simulink model "PRO_TestHarness"  (Simulink 8.6)
settings: Solver=ode45  StartTime=0.0  StopTime=10.0  RelTol=1e-3
PreLoadFcn:
  | addpath('./Workspace/')
  | load('./Workspace/EnvVar.mat')
  | if exist('tl_preloadfcn','file'), tl_preloadfcn(gcs,402); end
PostLoadFcn:
  | if exist('tl_postloadfcn','file'), tl_postloadfcn(gcs,402); end
InitFcn:
  | if exist('tlds_init','file'), tlds_init(gcs); end
StartFcn:
  | if exist('tlds_start','file'), tlds_start(gcs); end
StopFcn:
  | if exist('tlds_stop','file'), tlds_stop(gcs); end
undefined symbols (not defined in the file or in its folder): ddv, sigbuilder_block, Ts
libraries: tllib x19, simulink x2
(part 5 of 5)

== system PRO_TestHarness/PRO_AC_ProductionCycles/Subsystem/PRO_AC_ProductionCycles/PRO_AC_ProductionCycles/PRO_runProductionCycles/PRO enabled/FctTrigAbortCycle_AllPRO/For Iterator Subsystem/Algo PRO/FctTrigg_PRO ==
  bPreConditionsCommonFlag : Inport
  bPreActivation_PRO_in : Inport  Port=2
  Function : tllib/Function  data={'stepfunctionname','TriggerPRO','stepfunctionclass','STATIC_FCN_ASR4','codecomment',['This function is in charge of' char(10) 'providing the following outputs:' char(10) '' char(10) '- Trigger flag for PRO1 cycle' char(10) '- Pre Activation flag for PRO1 cycle' char(10) '- Pre Conditions flag for PRO1 cycle' char(10) '- Triggering Source for PRO1 cycle' char(10) '' char(10) 'according to the inputs:' char(10) '' char(10) '- executed cycle number' char(10) '- consistent cycle requested by diagnostic' char(10) '- common PRO preconditions flag'],'module','PRO_AC_ProductionCycles','date',736463.55395115737}  displayString=FUNCTION
  ToFormatFlag_PreActivationFlag : Subsystem
  ToFormatFlag_PreConditionsFlag : Subsystem
  ToFormatFlag_TriggeringOrder : Subsystem
  ToFormat_TriggeringSource : Subsystem
  bTriggeringOrder_Tester_PRO : Logic  AllPortsSameDT=off  OutDataTypeStr=boolean  mask(TL_LogicalOperator){data={'output',{'name','$B'},'date',735626.4046887384}}
      settings: DeleteFcn=if exist('delete_tlblock','file')==2,delete_tlblock(gcbh);end  NameChangeFcn=if exist('rename_tlblock','file')==2,rename_tlblock(gcbh);end  OpenFcn=if exist('tl_open_blockdlg','file')==2,tl_open_blockdlg(gcbh);else,open_system(gcbh,'parameter');end
      mask Help: eval(['if exist(''tl_online_help'',''file'') == 2, tl_online_help(''Topic'',''TL_LogicalOperator''),else, web([''jar:file:///'',matlabroot,''/help/toolbox/simulink/help.jar!/slref/' lower(get_param(gcbh,'Blocktype')) '.html''], ''-helpbrowser''),end'])
      mask Display: plot([-0.05, 1.05, NaN, -0.05, 1.05],[.01, .01, NaN, .99, .99])
  b8TriggeringOrder : Outport  PortDimensions=1
  b8PreActivationFlag : Outport  Port=2  PortDimensions=1
  b8PreConditionsFlag : Outport  Port=3  PortDimensions=1
  u8TriggeringSource_output : Outport  Port=4  PortDimensions=1
  wires:
  ToFormatFlag_TriggeringOrder/1(Out1) -> b8TriggeringOrder/1
  [bPreConditionsCommonFlag] -> ToFormatFlag_PreConditionsFlag/1(In1), bTriggeringOrder_Tester_PRO/1
  ToFormatFlag_PreConditionsFlag/1(Out1) -> b8PreConditionsFlag/1
  bTriggeringOrder_Tester_PRO/1 -> ToFormat_TriggeringSource/1(In1), ToFormatFlag_TriggeringOrder/1(In1)
  bPreConditionsCommonFlag/1 -> [bPreConditionsCommonFlag]
  ToFormatFlag_PreActivationFlag/1(Out2) -> b8PreActivationFlag/1
  ToFormat_TriggeringSource/1(Out1) -> u8TriggeringSource_output/1
  [bPreActivation_PRO] -> bTriggeringOrder_Tester_PRO/2
  [bPreActivation_PRO] -> ToFormatFlag_PreActivationFlag/1(In1)
  bPreActivation_PRO_in/1 -> [bPreActivation_PRO]

== system PRO_TestHarness/PRO_AC_ProductionCycles/Subsystem/PRO_AC_ProductionCycles/PRO_AC_ProductionCycles/PRO_runProductionCycles/PRO enabled/FctCommonPROManageInputs/FctCommonEvaluatePreActivationFlags/For Iterator Subsystem/FctEvaluatePreActivationFlags_PRO/Acquite Diag Request From DIA ==
  Action Port : ActionPort  ActionType=then
  ClearDiagRequestCycle : Subsystem  RequirementInfo={} %GIDa_6c044e8f_69a0_4de9_90b7_cd2120bfe9b6  TreatAsAtomicUnit=on

== system PRO_TestHarness/PRO_AC_ProductionCycles/Subsystem/PRO_AC_ProductionCycles/PRO_AC_ProductionCycles/PRO_runProductionCycles/PRO enabled/FctCommonPROManageInputs/FctCommonEvaluatePreActivationFlags/For Iterator Subsystem/FctEvaluatePreActivationFlags_PRO/Clear activation ==
  In1 : Inport
  Action Port : ActionPort  ActionType=elseif
  Out1 : Outport
  wires:
  In1/1 -> Out1/1

== system PRO_TestHarness/PRO_AC_ProductionCycles/Subsystem/PRO_AC_ProductionCycles/PRO_AC_ProductionCycles/PRO_runProductionCycles/PRO enabled/FctCommonPROManageInputs/FctCommonEvaluatePreActivationFlags/For Iterator Subsystem/FctEvaluatePreActivationFlags_PRO/Keep activation ==
  In1 : Inport
  Action Port : ActionPort  ActionType=else
  Out1 : Outport
  wires:
  In1/1 -> Out1/1

== system PRO_TestHarness/PRO_AC_ProductionCycles/Subsystem/PRO_AC_ProductionCycles/PRO_AC_ProductionCycles/PRO_runProductionCycles/PRO enabled/FctCommonPROManageInputs/FctCommonEvaluatePreActivationFlags/For Iterator Subsystem/FctEvaluatePreActivationFlags_PRO/Set activation ==
  In1 : Inport
  Action Port : ActionPort  ActionType=then
  Out1 : Outport
  wires:
  In1/1 -> Out1/1

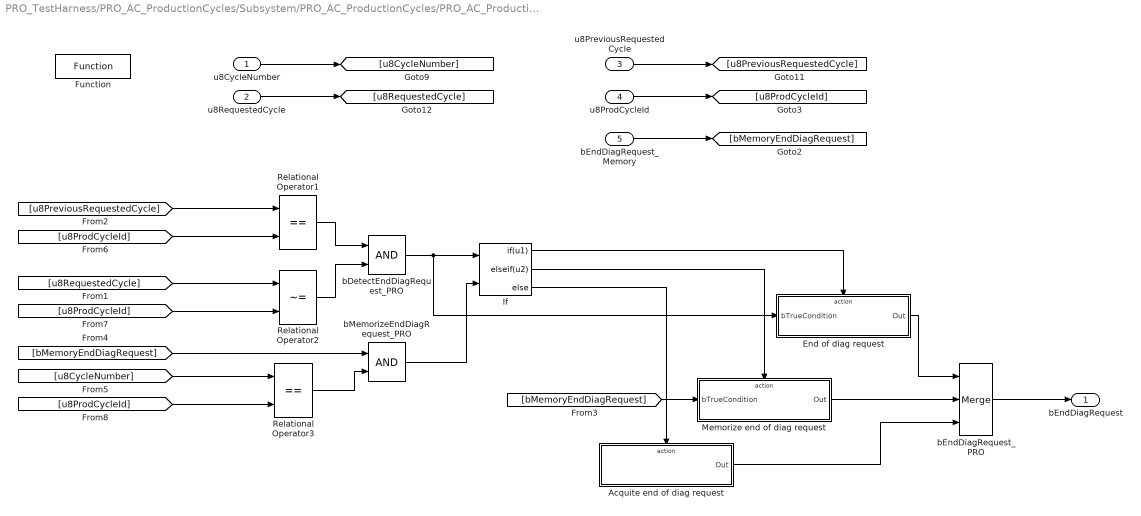
== system PRO_TestHarness/PRO_AC_ProductionCycles/Subsystem/PRO_AC_ProductionCycles/PRO_AC_ProductionCycles/PRO_runProductionCycles/PRO enabled/FctTrigAbortCycle_AllPRO/For Iterator Subsystem/Algo PRO/FctAbort_PRO/Check end diag request for PRO ==
  u8CycleNumber : Inport  PortDimensions=1
  u8RequestedCycle : Inport  Port=2  OutDataTypeStr=uint8  PortDimensions=1
  u8PreviousRequestedCycle : Inport  Port=3  OutDataTypeStr=uint8  PortDimensions=1
  u8ProdCycleId : Inport  Port=4  PortDimensions=1
  bEndDiagRequest_Memory : Inport  Port=5  PortDimensions=1
  Acquite end of diag request : Subsystem  TreatAsAtomicUnit=on
  End of diag request : Subsystem  TreatAsAtomicUnit=on
  Function : tllib/Function  data={'stepfunctionname','DetectEndOfDiagRequestPRO','stepfunctionclass','STATIC_FCN_ASR4','codecomment',['This function is in charge of' char(10) 'providing the following outputs:' char(10) '' char(10) '- End flag in case of PRO1 diagnostic request' char(10) '' char(10) 'according to the inputs:' char(10) '' char(10) '- executed cycle number' char(10) '- consistent cycle requested by diagnostic' char(10) '- previous (10 ms before) consistent cycle requested by diagnostic'],'module','PRO_AC_ProductionCycles','date',736463.55394269677}  displayString=FUNCTION
  If : If  NumInputs=2  IfExpression=u1  ElseIfExpressions=u2
  Memorize end of diag request : Subsystem  TreatAsAtomicUnit=on
  Relational Operator1 : RelationalOperator  Operator===  OutDataTypeStr=boolean  mask(TL_RelationalOperator){data={'date',735679.60375327547}}
      settings: DeleteFcn=if exist('delete_tlblock','file')==2,delete_tlblock(gcbh);end  NameChangeFcn=if exist('rename_tlblock','file')==2,rename_tlblock(gcbh);end  OpenFcn=if exist('tl_open_blockdlg','file')==2,tl_open_blockdlg(gcbh);else,open_system(gcbh,'parameter');end
      mask Help: eval(['if exist(''tl_online_help'',''file'') == 2, tl_online_help(''Topic'',''TL_RelationalOperator''),else, web([''jar:file:///'',matlabroot,''/help/toolbox/simulink/help.jar!/slref/' lower(get_param(gcbh,'Blocktype')) '.html''], ''-helpbrowser''),end'])
      mask Display: plot([-0.05, 1.05, NaN, -0.05, 1.05],[.01, .01, NaN, .99, .99])
  Relational Operator2 : RelationalOperator  Operator=~=  OutDataTypeStr=boolean  mask(TL_RelationalOperator){data={'date',735679.60375291668}}
      settings: DeleteFcn=if exist('delete_tlblock','file')==2,delete_tlblock(gcbh);end  NameChangeFcn=if exist('rename_tlblock','file')==2,rename_tlblock(gcbh);end  OpenFcn=if exist('tl_open_blockdlg','file')==2,tl_open_blockdlg(gcbh);else,open_system(gcbh,'parameter');end
      mask Help: eval(['if exist(''tl_online_help'',''file'') == 2, tl_online_help(''Topic'',''TL_RelationalOperator''),else, web([''jar:file:///'',matlabroot,''/help/toolbox/simulink/help.jar!/slref/' lower(get_param(gcbh,'Blocktype')) '.html''], ''-helpbrowser''),end'])
      mask Display: plot([-0.05, 1.05, NaN, -0.05, 1.05],[.01, .01, NaN, .99, .99])
  Relational Operator3 : RelationalOperator  Operator===  OutDataTypeStr=boolean  mask(TL_RelationalOperator){data={'date',735679.60375273146}}
      settings: DeleteFcn=if exist('delete_tlblock','file')==2,delete_tlblock(gcbh);end  NameChangeFcn=if exist('rename_tlblock','file')==2,rename_tlblock(gcbh);end  OpenFcn=if exist('tl_open_blockdlg','file')==2,tl_open_blockdlg(gcbh);else,open_system(gcbh,'parameter');end
      mask Help: eval(['if exist(''tl_online_help'',''file'') == 2, tl_online_help(''Topic'',''TL_RelationalOperator''),else, web([''jar:file:///'',matlabroot,''/help/toolbox/simulink/help.jar!/slref/' lower(get_param(gcbh,'Blocktype')) '.html''], ''-helpbrowser''),end'])
      mask Display: plot([-0.05, 1.05, NaN, -0.05, 1.05],[.01, .01, NaN, .99, .99])
  bDetectEndDiagRequest_PRO : Logic  AllPortsSameDT=off  OutDataTypeStr=boolean  mask(TL_LogicalOperator){data={'output',{'name','$B'},'date',735679.60375237267}}
      settings: DeleteFcn=if exist('delete_tlblock','file')==2,delete_tlblock(gcbh);end  NameChangeFcn=if exist('rename_tlblock','file')==2,rename_tlblock(gcbh);end  OpenFcn=if exist('tl_open_blockdlg','file')==2,tl_open_blockdlg(gcbh);else,open_system(gcbh,'parameter');end
      mask Help: eval(['if exist(''tl_online_help'',''file'') == 2, tl_online_help(''Topic'',''TL_LogicalOperator''),else, web([''jar:file:///'',matlabroot,''/help/toolbox/simulink/help.jar!/slref/' lower(get_param(gcbh,'Blocktype')) '.html''], ''-helpbrowser''),end'])
      mask Display: plot([-0.05, 1.05, NaN, -0.05, 1.05],[.01, .01, NaN, .99, .99])
  bEndDiagRequest_PRO : Merge  Inputs=3  InitialOutput=0  mask(TL_Merge){data={'output',{'name','$B','type','Bool','inheritscaling',0},'date',735679.60375219909}}
      settings: CopyFcn=if exist('tl_reset_reviewflag','file')==2,tl_reset_reviewflag(gcbh);end  DeleteFcn=if exist('delete_tlblock','file')==2,delete_tlblock(gcbh);end  NameChangeFcn=if exist('rename_tlblock','file')==2,rename_tlblock(gcbh);end  OpenFcn=if exist('tl_open_blockdlg','file')==2,tl_open_blockdlg(gcbh);else,open_system(gcbh,'parameter');end
      mask Help: eval(['if exist(''tl_online_help'',''file'') == 2, tl_online_help(''Topic'',''TL_Merge''),else, web([''jar:file:///'',matlabroot,''/help/toolbox/simulink/help.jar!/slref/' lower(get_param(gcbh,'Blocktype')) '.html''], ''-helpbrowser''),end'])
      mask Display: plot([-0.05, 1.05, NaN, -0.05, 1.05],[.01, .01, NaN, .99, .99])
  bMemorizeEndDiagRequest_PRO : Logic  AllPortsSameDT=off  OutDataTypeStr=boolean  mask(TL_LogicalOperator){data={'output',{'name','$B'},'date',735679.60375165509}}
      settings: DeleteFcn=if exist('delete_tlblock','file')==2,delete_tlblock(gcbh);end  NameChangeFcn=if exist('rename_tlblock','file')==2,rename_tlblock(gcbh);end  OpenFcn=if exist('tl_open_blockdlg','file')==2,tl_open_blockdlg(gcbh);else,open_system(gcbh,'parameter');end
      mask Help: eval(['if exist(''tl_online_help'',''file'') == 2, tl_online_help(''Topic'',''TL_LogicalOperator''),else, web([''jar:file:///'',matlabroot,''/help/toolbox/simulink/help.jar!/slref/' lower(get_param(gcbh,'Blocktype')) '.html''], ''-helpbrowser''),end'])
      mask Display: plot([-0.05, 1.05, NaN, -0.05, 1.05],[.01, .01, NaN, .99, .99])
  bEndDiagRequest : Outport  PortDimensions=1
  wires:
  [u8ProdCycleId] -> Relational Operator1/2
  [u8PreviousRequestedCycle] -> Relational Operator1/1
  Relational Operator1/1 -> bDetectEndDiagRequest_PRO/1
  [u8RequestedCycle] -> Relational Operator2/1
  [u8ProdCycleId] -> Relational Operator2/2
  Relational Operator2/1 -> bDetectEndDiagRequest_PRO/2
  bDetectEndDiagRequest_PRO/1 -> If/1, End of diag request/1(bTrueCondition)
  If/1 -> End of diag request/Action
  End of diag request/1(Out) -> bEndDiagRequest_PRO/1
  Memorize end of diag request/1(Out) -> bEndDiagRequest_PRO/2
  Acquite end of diag request/1(Out) -> bEndDiagRequest_PRO/3
  If/2 -> Memorize end of diag request/Action
  If/3 -> Acquite end of diag request/Action
  [bMemoryEndDiagRequest] -> Memorize end of diag request/1(bTrueCondition)
  [u8CycleNumber] -> Relational Operator3/1
  [u8ProdCycleId] -> Relational Operator3/2
  [bMemoryEndDiagRequest] -> bMemorizeEndDiagRequest_PRO/1
  bMemorizeEndDiagRequest_PRO/1 -> If/2
  Relational Operator3/1 -> bMemorizeEndDiagRequest_PRO/2
  bEndDiagRequest_PRO/1 -> bEndDiagRequest/1
  u8CycleNumber/1 -> [u8CycleNumber]
  u8RequestedCycle/1 -> [u8RequestedCycle]
  u8PreviousRequestedCycle/1 -> [u8PreviousRequestedCycle]
  u8ProdCycleId/1 -> [u8ProdCycleId]
  bEndDiagRequest_Memory/1 -> [bMemoryEndDiagRequest]

== system PRO_TestHarness/PRO_AC_ProductionCycles/Subsystem/PRO_AC_ProductionCycles/PRO_AC_ProductionCycles/PRO_runProductionCycles/PRO enabled/FctTrigAbortCycle_AllPRO/For Iterator Subsystem/Algo PRO/FctAbort_PRO/ToFormatFlag_bInterruptFlag ==
  In1 : Inport
  If Action Subsystem4 : Subsystem  TreatAsAtomicUnit=on
  If Action Subsystem5 : Subsystem  TreatAsAtomicUnit=on
  If2 : If  IfExpression=u1
  b8ComputedInterruptFlag : Merge  InitialOutput=[ddv('RTE_DEFINES/KB8_ALGO_FLAG_OFF')]  mask(TL_Merge){data={'output',{'type','UInt8','inheritscaling',0},'date',736811.34356223384}}
      settings: CopyFcn=if exist('tl_reset_reviewflag') == 2, tl_reset_reviewflag(gcbh); end  DeleteFcn=if exist('delete_tlblock','file')==2,delete_tlblock(gcbh);end  NameChangeFcn=if exist('rename_tlblock','file')==2,rename_tlblock(gcbh);end  OpenFcn=if exist('tl_open_blockdlg','file')==2,tl_open_blockdlg(gcbh);else,open_system(gcbh,'parameter');end
      mask Help: eval(['if exist(''tl_online_help'',''file'') == 2, tl_online_help(''Topic'',''TL_Merge''),else, web([''jar:file:///'',matlabroot,''/help/toolbox/simulink/help.jar!/slref/' lower(get_param(gcbh,'Blocktype')) '.html''], ''-helpbrowser''),end'])
      mask Display: plot([-0.05, 1.05, NaN, -0.05, 1.05],[.01, .01, NaN, .99, .99])
  b8NewInterruptFlag_PRO : Gain  OutDataTypeStr=uint8  mask(TL_Gain){data={'output',{'name','$B','type','UInt8'},'date',735664.46096548613}}
      settings: CopyFcn=if exist('tl_reset_reviewflag') == 2, tl_reset_reviewflag(gcbh); end  DeleteFcn=if exist('delete_tlblock','file')==2,delete_tlblock(gcbh);end  NameChangeFcn=if exist('rename_tlblock','file')==2,rename_tlblock(gcbh);end  OpenFcn=if exist('tl_open_blockdlg','file')==2,tl_open_blockdlg(gcbh);else,open_system(gcbh,'parameter');end
      mask Help: eval(['if exist(''tl_online_help'',''file'') == 2, tl_online_help(''Topic'',''TL_Gain''),else, web([''jar:file:///'',matlabroot,''/help/toolbox/simulink/help.jar!/slref/' lower(get_param(gcbh,'Blocktype')) '.html''], ''-helpbrowser''),end'])
      mask Display: plot([0, .9, 0],[.05, .5, .95])
  Out1 : Outport
  wires:
  If2/1 -> If Action Subsystem4/Action
  b8ComputedInterruptFlag/1 -> b8NewInterruptFlag_PRO/1
  If Action Subsystem4/1(Out) -> b8ComputedInterruptFlag/1
  If Action Subsystem5/1(Out) -> b8ComputedInterruptFlag/2
  If2/2 -> If Action Subsystem5/Action
  In1/1 -> If2/1
  b8NewInterruptFlag_PRO/1 -> Out1/1

== system PRO_TestHarness/PRO_AC_ProductionCycles/Subsystem/PRO_AC_ProductionCycles/PRO_AC_ProductionCycles/PRO_runProductionCycles/PRO enabled/FctTrigAbortCycle_AllPRO/For Iterator Subsystem/Algo PRO/FctTrigg_PRO/ToFormatFlag_PreActivationFlag ==
  In1 : Inport
  If : If  IfExpression=u1
  If Action Subsystem : Subsystem  TreatAsAtomicUnit=on
  If Action Subsystem1 : Subsystem  TreatAsAtomicUnit=on
  b8NewPreActivationFlag_PRO : Gain  OutDataTypeStr=uint8  mask(TL_Gain){data={'output',{'name','$B','type','UInt8'},'date',735661.6408991667}}
      settings: CopyFcn=if exist('tl_reset_reviewflag') == 2, tl_reset_reviewflag(gcbh); end  DeleteFcn=if exist('delete_tlblock','file')==2,delete_tlblock(gcbh);end  NameChangeFcn=if exist('rename_tlblock','file')==2,rename_tlblock(gcbh);end  OpenFcn=if exist('tl_open_blockdlg','file')==2,tl_open_blockdlg(gcbh);else,open_system(gcbh,'parameter');end
      mask Help: eval(['if exist(''tl_online_help'',''file'') == 2, tl_online_help(''Topic'',''TL_Gain''),else, web([''jar:file:///'',matlabroot,''/help/toolbox/simulink/help.jar!/slref/' lower(get_param(gcbh,'Blocktype')) '.html''], ''-helpbrowser''),end'])
      mask Display: plot([0, .9, 0],[.05, .5, .95])
  b8PreActivationFlag_PRO : Merge  InitialOutput=[ddv('RTE_DEFINES/KB8_ALGO_FLAG_OFF')]  mask(TL_Merge){data={'output',{'type','UInt8','inheritscaling',0},'date',736811.34117243055}}
      settings: CopyFcn=if exist('tl_reset_reviewflag') == 2, tl_reset_reviewflag(gcbh); end  DeleteFcn=if exist('delete_tlblock','file')==2,delete_tlblock(gcbh);end  NameChangeFcn=if exist('rename_tlblock','file')==2,rename_tlblock(gcbh);end  OpenFcn=if exist('tl_open_blockdlg','file')==2,tl_open_blockdlg(gcbh);else,open_system(gcbh,'parameter');end
      mask Help: eval(['if exist(''tl_online_help'',''file'') == 2, tl_online_help(''Topic'',''TL_Merge''),else, web([''jar:file:///'',matlabroot,''/help/toolbox/simulink/help.jar!/slref/' lower(get_param(gcbh,'Blocktype')) '.html''], ''-helpbrowser''),end'])
      mask Display: plot([-0.05, 1.05, NaN, -0.05, 1.05],[.01, .01, NaN, .99, .99])
  Out2 : Outport
  wires:
  If/1 -> If Action Subsystem/Action
  b8PreActivationFlag_PRO/1 -> b8NewPreActivationFlag_PRO/1
  If Action Subsystem/1(Out) -> b8PreActivationFlag_PRO/1
  If Action Subsystem1/1(Out) -> b8PreActivationFlag_PRO/2
  If/2 -> If Action Subsystem1/Action
  In1/1 -> If/1
  b8NewPreActivationFlag_PRO/1 -> Out2/1

== system PRO_TestHarness/PRO_AC_ProductionCycles/Subsystem/PRO_AC_ProductionCycles/PRO_AC_ProductionCycles/PRO_runProductionCycles/PRO enabled/FctTrigAbortCycle_AllPRO/For Iterator Subsystem/Algo PRO/FctTrigg_PRO/ToFormatFlag_PreConditionsFlag ==
  In1 : Inport
  If Action Subsystem4 : Subsystem  TreatAsAtomicUnit=on
  If Action Subsystem5 : Subsystem  TreatAsAtomicUnit=on
  If2 : If  IfExpression=u1
  b8ComputedPreConditionsFlag : Merge  InitialOutput=[ddv('RTE_DEFINES/KB8_ALGO_FLAG_OFF')]  mask(TL_Merge){data={'output',{'type','UInt8','inheritscaling',0},'date',736811.341286632}}
      settings: CopyFcn=if exist('tl_reset_reviewflag') == 2, tl_reset_reviewflag(gcbh); end  DeleteFcn=if exist('delete_tlblock','file')==2,delete_tlblock(gcbh);end  NameChangeFcn=if exist('rename_tlblock','file')==2,rename_tlblock(gcbh);end  OpenFcn=if exist('tl_open_blockdlg','file')==2,tl_open_blockdlg(gcbh);else,open_system(gcbh,'parameter');end
      mask Help: eval(['if exist(''tl_online_help'',''file'') == 2, tl_online_help(''Topic'',''TL_Merge''),else, web([''jar:file:///'',matlabroot,''/help/toolbox/simulink/help.jar!/slref/' lower(get_param(gcbh,'Blocktype')) '.html''], ''-helpbrowser''),end'])
      mask Display: plot([-0.05, 1.05, NaN, -0.05, 1.05],[.01, .01, NaN, .99, .99])
  b8NewPreConditionsFlag_PRO : Gain  OutDataTypeStr=uint8  mask(TL_Gain){data={'output',{'name','$B','type','UInt8'},'date',735661.64106355328}}
      settings: CopyFcn=if exist('tl_reset_reviewflag') == 2, tl_reset_reviewflag(gcbh); end  DeleteFcn=if exist('delete_tlblock','file')==2,delete_tlblock(gcbh);end  NameChangeFcn=if exist('rename_tlblock','file')==2,rename_tlblock(gcbh);end  OpenFcn=if exist('tl_open_blockdlg','file')==2,tl_open_blockdlg(gcbh);else,open_system(gcbh,'parameter');end
      mask Help: eval(['if exist(''tl_online_help'',''file'') == 2, tl_online_help(''Topic'',''TL_Gain''),else, web([''jar:file:///'',matlabroot,''/help/toolbox/simulink/help.jar!/slref/' lower(get_param(gcbh,'Blocktype')) '.html''], ''-helpbrowser''),end'])
      mask Display: plot([0, .9, 0],[.05, .5, .95])
  Out1 : Outport
  wires:
  If2/1 -> If Action Subsystem4/Action
  b8ComputedPreConditionsFlag/1 -> b8NewPreConditionsFlag_PRO/1
  If Action Subsystem4/1(Out) -> b8ComputedPreConditionsFlag/1
  If Action Subsystem5/1(Out) -> b8ComputedPreConditionsFlag/2
  If2/2 -> If Action Subsystem5/Action
  In1/1 -> If2/1
  b8NewPreConditionsFlag_PRO/1 -> Out1/1

== system PRO_TestHarness/PRO_AC_ProductionCycles/Subsystem/PRO_AC_ProductionCycles/PRO_AC_ProductionCycles/PRO_runProductionCycles/PRO enabled/FctTrigAbortCycle_AllPRO/For Iterator Subsystem/Algo PRO/FctTrigg_PRO/ToFormatFlag_TriggeringOrder ==
  In1 : Inport
  If : If  IfExpression=u1
  If Action Subsystem : Subsystem  TreatAsAtomicUnit=on
  If Action Subsystem1 : Subsystem  TreatAsAtomicUnit=on
  b8ComputedTriggeringOrder : Merge  InitialOutput=[ddv('RTE_DEFINES/KB8_ALGO_FLAG_OFF')]  mask(TL_Merge){data={'output',{'type','UInt8','inheritscaling',0},'date',736811.3418450926}}
      settings: CopyFcn=if exist('tl_reset_reviewflag') == 2, tl_reset_reviewflag(gcbh); end  DeleteFcn=if exist('delete_tlblock','file')==2,delete_tlblock(gcbh);end  NameChangeFcn=if exist('rename_tlblock','file')==2,rename_tlblock(gcbh);end  OpenFcn=if exist('tl_open_blockdlg','file')==2,tl_open_blockdlg(gcbh);else,open_system(gcbh,'parameter');end
      mask Help: eval(['if exist(''tl_online_help'',''file'') == 2, tl_online_help(''Topic'',''TL_Merge''),else, web([''jar:file:///'',matlabroot,''/help/toolbox/simulink/help.jar!/slref/' lower(get_param(gcbh,'Blocktype')) '.html''], ''-helpbrowser''),end'])
      mask Display: plot([-0.05, 1.05, NaN, -0.05, 1.05],[.01, .01, NaN, .99, .99])
  b8NewTriggeringOrder_PRO : Gain  OutDataTypeStr=uint8  mask(TL_Gain){data={'output',{'name','$B','type','UInt8'},'date',735661.6408991667}}
      settings: CopyFcn=if exist('tl_reset_reviewflag') == 2, tl_reset_reviewflag(gcbh); end  DeleteFcn=if exist('delete_tlblock','file')==2,delete_tlblock(gcbh);end  NameChangeFcn=if exist('rename_tlblock','file')==2,rename_tlblock(gcbh);end  OpenFcn=if exist('tl_open_blockdlg','file')==2,tl_open_blockdlg(gcbh);else,open_system(gcbh,'parameter');end
      mask Help: eval(['if exist(''tl_online_help'',''file'') == 2, tl_online_help(''Topic'',''TL_Gain''),else, web([''jar:file:///'',matlabroot,''/help/toolbox/simulink/help.jar!/slref/' lower(get_param(gcbh,'Blocktype')) '.html''], ''-helpbrowser''),end'])
      mask Display: plot([0, .9, 0],[.05, .5, .95])
  Out1 : Outport
  wires:
  If/1 -> If Action Subsystem/Action
  b8ComputedTriggeringOrder/1 -> b8NewTriggeringOrder_PRO/1
  If Action Subsystem/1(Out) -> b8ComputedTriggeringOrder/1
  If Action Subsystem1/1(Out) -> b8ComputedTriggeringOrder/2
  If/2 -> If Action Subsystem1/Action
  In1/1 -> If/1
  b8NewTriggeringOrder_PRO/1 -> Out1/1

== system PRO_TestHarness/PRO_AC_ProductionCycles/Subsystem/PRO_AC_ProductionCycles/PRO_AC_ProductionCycles/PRO_runProductionCycles/PRO enabled/FctTrigAbortCycle_AllPRO/For Iterator Subsystem/Algo PRO/FctTrigg_PRO/ToFormat_TriggeringSource ==
  In1 : Inport
  If3 : If  IfExpression=u1
  None : Subsystem  TreatAsAtomicUnit=on
  Tester : Subsystem  TreatAsAtomicUnit=on
  u8NewTriggeringSource_PRO : Gain  OutDataTypeStr=uint8  mask(TL_Gain){data={'output',{'name','$B','type','UInt8'},'date',735402.45745033561}}
      settings: CopyFcn=if exist('tl_reset_reviewflag') == 2, tl_reset_reviewflag(gcbh); end  DeleteFcn=if exist('delete_tlblock','file')==2,delete_tlblock(gcbh);end  NameChangeFcn=if exist('rename_tlblock','file')==2,rename_tlblock(gcbh);end  OpenFcn=if exist('tl_open_blockdlg','file')==2,tl_open_blockdlg(gcbh);else,open_system(gcbh,'parameter');end
      mask Help: eval(['if exist(''tl_online_help'',''file'') == 2, tl_online_help(''Topic'',''TL_Gain''),else, web([''jar:file:///'',matlabroot,''/help/toolbox/simulink/help.jar!/slref/' lower(get_param(gcbh,'Blocktype')) '.html''], ''-helpbrowser''),end'])
      mask Display: plot([0, .9, 0],[.05, .5, .95])
  u8TriggeringSource_PRO : Merge  InitialOutput=[ddv('RTE_DEFINES/KB8_ALGO_FLAG_OFF')]  mask(TL_Merge){data={'output',{'name','$B','type','UInt8','inheritscaling',0},'date',736811.34286805557}}
      settings: CopyFcn=if exist('tl_reset_reviewflag') == 2, tl_reset_reviewflag(gcbh); end  DeleteFcn=if exist('delete_tlblock','file')==2,delete_tlblock(gcbh);end  NameChangeFcn=if exist('rename_tlblock','file')==2,rename_tlblock(gcbh);end  OpenFcn=if exist('tl_open_blockdlg','file')==2,tl_open_blockdlg(gcbh);else,open_system(gcbh,'parameter');end
      mask Help: eval(['if exist(''tl_online_help'',''file'') == 2, tl_online_help(''Topic'',''TL_Merge''),else, web([''jar:file:///'',matlabroot,''/help/toolbox/simulink/help.jar!/slref/' lower(get_param(gcbh,'Blocktype')) '.html''], ''-helpbrowser''),end'])
      mask Display: plot([-0.05, 1.05, NaN, -0.05, 1.05],[.01, .01, NaN, .99, .99])
  Out1 : Outport
  wires:
  u8TriggeringSource_PRO/1 -> u8NewTriggeringSource_PRO/1
  If3/2 -> None/Action
  u8NewTriggeringSource_PRO/1 -> Out1/1
  Tester/1(u8TriggeringSource) -> u8TriggeringSource_PRO/1
  If3/1 -> Tester/Action
  None/1(u8TriggeringSource) -> u8TriggeringSource_PRO/2
  In1/1 -> If3/1

== system PRO_TestHarness/PRO_AC_ProductionCycles/Subsystem/PRO_AC_ProductionCycles/PRO_AC_ProductionCycles/PRO_runProductionCycles/PRO enabled/FctCommonPROManageInputs/FctCommonEvaluatePreActivationFlags/For Iterator Subsystem/FctEvaluatePreActivationFlags_PRO/Acquite Diag Request From DIA/ClearDiagRequestCycle ==
  Inserted Function block : tllib/Function  RequirementInfo={} %GIDa_6b54e211_970f_4d53_9b14_76c85f7e42ac  data={'stepfunctionclass','STATIC_FCN_ASR4','autosar',{'useautosarspecification',1,'functionrole',3,'clientport','pclDiagRequestCycle','operation','ClearDiagRequestCycle','isimplementationforsilpil',0,'clientsoftwarecomponent','AUTOLIV/SoftwareComponents/PRO/PRO_AC_ProductionCycles'},'date',736811.32660879625}  displayString=|
      | OPERATION CALL
      | (SYNCHRONOUS)

== system PRO_TestHarness/PRO_AC_ProductionCycles/Subsystem/PRO_AC_ProductionCycles/PRO_AC_ProductionCycles/PRO_runProductionCycles/PRO enabled/FctTrigAbortCycle_AllPRO/For Iterator Subsystem/Algo PRO/FctAbort_PRO/Check end diag request for PRO/Acquite end of diag request ==
  Action Port : ActionPort  ActionType=else
  Constant5 : Constant  Value=ddv('BFD/KB_ZERO')  OutDataTypeStr=boolean  mask(TL_Constant){data={'output',{'variable','BFD/KB_ZERO'},'date',735679.61958113429}}
      settings: CopyFcn=if exist('tl_reset_reviewflag','file')==2,tl_reset_reviewflag(gcbh);end  DeleteFcn=if exist('delete_tlblock','file')==2,delete_tlblock(gcbh);end  NameChangeFcn=if exist('rename_tlblock','file')==2,rename_tlblock(gcbh);end  OpenFcn=if exist('tl_open_blockdlg','file')==2,tl_open_blockdlg(gcbh);else,open_system(gcbh,'parameter');end
      mask Help: eval(['if exist(''tl_online_help'',''file'') == 2, tl_online_help(''Topic'',''TL_Constant''),else, web([''jar:file:///'',matlabroot,''/help/toolbox/simulink/help.jar!/slref/' lower(get_param(gcbh,'Blocktype')) '.html''], ''-helpbrowser''),end'])
      mask Display: plot([-0.05, 1.05, NaN, -0.05, 1.05],[.01, .01, NaN, .99, .99])
  Out : Outport  PortDimensions=1  InitialOutput=[0]
  wires:
  Constant5/1 -> Out/1

== system PRO_TestHarness/PRO_AC_ProductionCycles/Subsystem/PRO_AC_ProductionCycles/PRO_AC_ProductionCycles/PRO_runProductionCycles/PRO enabled/FctTrigAbortCycle_AllPRO/For Iterator Subsystem/Algo PRO/FctAbort_PRO/Check end diag request for PRO/End of diag request ==
  bTrueCondition : Inport
  Action Port : ActionPort  ActionType=then
  Out : Outport  PortDimensions=1  InitialOutput=[0]
  wires:
  bTrueCondition/1 -> Out/1

== system PRO_TestHarness/PRO_AC_ProductionCycles/Subsystem/PRO_AC_ProductionCycles/PRO_AC_ProductionCycles/PRO_runProductionCycles/PRO enabled/FctTrigAbortCycle_AllPRO/For Iterator Subsystem/Algo PRO/FctAbort_PRO/Check end diag request for PRO/Memorize end of diag request ==
  bTrueCondition : Inport
  Action Port : ActionPort  ActionType=elseif
  Out : Outport  PortDimensions=1  InitialOutput=[0]
  wires:
  bTrueCondition/1 -> Out/1

== system PRO_TestHarness/PRO_AC_ProductionCycles/Subsystem/PRO_AC_ProductionCycles/PRO_AC_ProductionCycles/PRO_runProductionCycles/PRO enabled/FctTrigAbortCycle_AllPRO/For Iterator Subsystem/Algo PRO/FctAbort_PRO/ToFormatFlag_bInterruptFlag/If Action Subsystem4 ==
  Action Port : ActionPort  ActionType=then
  Constant1 : Constant  Value=ddv('RTE_DEFINES/KB8_ALGO_FLAG_ON')  OutDataTypeStr=uint8  mask(TL_Constant){data={'output',{'variable','RTE_DEFINES/KB8_ALGO_FLAG_ON'},'date',736811.34363208339}}
      settings: DeleteFcn=if exist('delete_tlblock','file')==2,delete_tlblock(gcbh);end  NameChangeFcn=if exist('rename_tlblock','file')==2,rename_tlblock(gcbh);end  OpenFcn=if exist('tl_open_blockdlg','file')==2,tl_open_blockdlg(gcbh);else,open_system(gcbh,'parameter');end
      mask Help: eval(['if exist(''tl_online_help'',''file'') == 2, tl_online_help(''Topic'',''TL_Constant''),else, web([''jar:file:///'',matlabroot,''/help/toolbox/simulink/help.jar!/slref/' lower(get_param(gcbh,'Blocktype')) '.html''], ''-helpbrowser''),end'])
      mask Display: plot([-0.05, 1.05, NaN, -0.05, 1.05],[.01, .01, NaN, .99, .99])
  Out : Outport  PortDimensions=1  InitialOutput=[0]
  wires:
  Constant1/1 -> Out/1

== system PRO_TestHarness/PRO_AC_ProductionCycles/Subsystem/PRO_AC_ProductionCycles/PRO_AC_ProductionCycles/PRO_runProductionCycles/PRO enabled/FctTrigAbortCycle_AllPRO/For Iterator Subsystem/Algo PRO/FctAbort_PRO/ToFormatFlag_bInterruptFlag/If Action Subsystem5 ==
  Action Port : ActionPort  ActionType=else
  Constant1 : Constant  Value=ddv('RTE_DEFINES/KB8_ALGO_FLAG_OFF')  OutDataTypeStr=uint8  mask(TL_Constant){data={'output',{'variable','RTE_DEFINES/KB8_ALGO_FLAG_OFF'},'date',736811.34373133106}}
      settings: DeleteFcn=if exist('delete_tlblock','file')==2,delete_tlblock(gcbh);end  NameChangeFcn=if exist('rename_tlblock','file')==2,rename_tlblock(gcbh);end  OpenFcn=if exist('tl_open_blockdlg','file')==2,tl_open_blockdlg(gcbh);else,open_system(gcbh,'parameter');end
      mask Help: eval(['if exist(''tl_online_help'',''file'') == 2, tl_online_help(''Topic'',''TL_Constant''),else, web([''jar:file:///'',matlabroot,''/help/toolbox/simulink/help.jar!/slref/' lower(get_param(gcbh,'Blocktype')) '.html''], ''-helpbrowser''),end'])
      mask Display: plot([-0.05, 1.05, NaN, -0.05, 1.05],[.01, .01, NaN, .99, .99])
  Out : Outport  PortDimensions=1  InitialOutput=[0]
  wires:
  Constant1/1 -> Out/1

== system PRO_TestHarness/PRO_AC_ProductionCycles/Subsystem/PRO_AC_ProductionCycles/PRO_AC_ProductionCycles/PRO_runProductionCycles/PRO enabled/FctTrigAbortCycle_AllPRO/For Iterator Subsystem/Algo PRO/FctTrigg_PRO/ToFormatFlag_PreActivationFlag/If Action Subsystem ==
  Action Port : ActionPort  ActionType=then
  Constant1 : Constant  Value=ddv('RTE_DEFINES/KB8_ALGO_FLAG_ON')  OutDataTypeStr=uint8  mask(TL_Constant){data={'output',{'variable','RTE_DEFINES/KB8_ALGO_FLAG_ON'},'date',736811.34088271996}}
      settings: DeleteFcn=if exist('delete_tlblock','file')==2,delete_tlblock(gcbh);end  NameChangeFcn=if exist('rename_tlblock','file')==2,rename_tlblock(gcbh);end  OpenFcn=if exist('tl_open_blockdlg','file')==2,tl_open_blockdlg(gcbh);else,open_system(gcbh,'parameter');end
      mask Help: eval(['if exist(''tl_online_help'',''file'') == 2, tl_online_help(''Topic'',''TL_Constant''),else, web([''jar:file:///'',matlabroot,''/help/toolbox/simulink/help.jar!/slref/' lower(get_param(gcbh,'Blocktype')) '.html''], ''-helpbrowser''),end'])
      mask Display: plot([-0.05, 1.05, NaN, -0.05, 1.05],[.01, .01, NaN, .99, .99])
  Out : Outport  PortDimensions=1  InitialOutput=[0]
  wires:
  Constant1/1 -> Out/1

== system PRO_TestHarness/PRO_AC_ProductionCycles/Subsystem/PRO_AC_ProductionCycles/PRO_AC_ProductionCycles/PRO_runProductionCycles/PRO enabled/FctTrigAbortCycle_AllPRO/For Iterator Subsystem/Algo PRO/FctTrigg_PRO/ToFormatFlag_PreActivationFlag/If Action Subsystem1 ==
  Action Port : ActionPort  ActionType=else
  Constant1 : Constant  Value=ddv('RTE_DEFINES/KB8_ALGO_FLAG_OFF')  OutDataTypeStr=uint8  mask(TL_Constant){data={'output',{'variable','RTE_DEFINES/KB8_ALGO_FLAG_OFF'},'date',736811.34103421296}}
      settings: DeleteFcn=if exist('delete_tlblock','file')==2,delete_tlblock(gcbh);end  NameChangeFcn=if exist('rename_tlblock','file')==2,rename_tlblock(gcbh);end  OpenFcn=if exist('tl_open_blockdlg','file')==2,tl_open_blockdlg(gcbh);else,open_system(gcbh,'parameter');end
      mask Help: eval(['if exist(''tl_online_help'',''file'') == 2, tl_online_help(''Topic'',''TL_Constant''),else, web([''jar:file:///'',matlabroot,''/help/toolbox/simulink/help.jar!/slref/' lower(get_param(gcbh,'Blocktype')) '.html''], ''-helpbrowser''),end'])
      mask Display: plot([-0.05, 1.05, NaN, -0.05, 1.05],[.01, .01, NaN, .99, .99])
  Out : Outport  PortDimensions=1  InitialOutput=[0]
  wires:
  Constant1/1 -> Out/1

== system PRO_TestHarness/PRO_AC_ProductionCycles/Subsystem/PRO_AC_ProductionCycles/PRO_AC_ProductionCycles/PRO_runProductionCycles/PRO enabled/FctTrigAbortCycle_AllPRO/For Iterator Subsystem/Algo PRO/FctTrigg_PRO/ToFormatFlag_PreConditionsFlag/If Action Subsystem4 ==
  Action Port : ActionPort  ActionType=then
  Constant1 : Constant  Value=ddv('RTE_DEFINES/KB8_ALGO_FLAG_ON')  OutDataTypeStr=uint8  mask(TL_Constant){data={'output',{'variable','RTE_DEFINES/KB8_ALGO_FLAG_ON'},'date',736811.34136861109}}
      settings: DeleteFcn=if exist('delete_tlblock','file')==2,delete_tlblock(gcbh);end  NameChangeFcn=if exist('rename_tlblock','file')==2,rename_tlblock(gcbh);end  OpenFcn=if exist('tl_open_blockdlg','file')==2,tl_open_blockdlg(gcbh);else,open_system(gcbh,'parameter');end
      mask Help: eval(['if exist(''tl_online_help'',''file'') == 2, tl_online_help(''Topic'',''TL_Constant''),else, web([''jar:file:///'',matlabroot,''/help/toolbox/simulink/help.jar!/slref/' lower(get_param(gcbh,'Blocktype')) '.html''], ''-helpbrowser''),end'])
      mask Display: plot([-0.05, 1.05, NaN, -0.05, 1.05],[.01, .01, NaN, .99, .99])
  Out : Outport  PortDimensions=1  InitialOutput=[0]
  wires:
  Constant1/1 -> Out/1

== system PRO_TestHarness/PRO_AC_ProductionCycles/Subsystem/PRO_AC_ProductionCycles/PRO_AC_ProductionCycles/PRO_runProductionCycles/PRO enabled/FctTrigAbortCycle_AllPRO/For Iterator Subsystem/Algo PRO/FctTrigg_PRO/ToFormatFlag_PreConditionsFlag/If Action Subsystem5 ==
  Action Port : ActionPort  ActionType=else
  Constant1 : Constant  Value=ddv('RTE_DEFINES/KB8_ALGO_FLAG_OFF')  OutDataTypeStr=uint8  mask(TL_Constant){data={'output',{'variable','RTE_DEFINES/KB8_ALGO_FLAG_OFF'},'date',736811.34154383105}}
      settings: DeleteFcn=if exist('delete_tlblock','file')==2,delete_tlblock(gcbh);end  NameChangeFcn=if exist('rename_tlblock','file')==2,rename_tlblock(gcbh);end  OpenFcn=if exist('tl_open_blockdlg','file')==2,tl_open_blockdlg(gcbh);else,open_system(gcbh,'parameter');end
      mask Help: eval(['if exist(''tl_online_help'',''file'') == 2, tl_online_help(''Topic'',''TL_Constant''),else, web([''jar:file:///'',matlabroot,''/help/toolbox/simulink/help.jar!/slref/' lower(get_param(gcbh,'Blocktype')) '.html''], ''-helpbrowser''),end'])
      mask Display: plot([-0.05, 1.05, NaN, -0.05, 1.05],[.01, .01, NaN, .99, .99])
  Out : Outport  PortDimensions=1  InitialOutput=[0]
  wires:
  Constant1/1 -> Out/1

== system PRO_TestHarness/PRO_AC_ProductionCycles/Subsystem/PRO_AC_ProductionCycles/PRO_AC_ProductionCycles/PRO_runProductionCycles/PRO enabled/FctTrigAbortCycle_AllPRO/For Iterator Subsystem/Algo PRO/FctTrigg_PRO/ToFormatFlag_TriggeringOrder/If Action Subsystem ==
  Action Port : ActionPort  ActionType=then
  Constant1 : Constant  Value=ddv('RTE_DEFINES/KB8_ALGO_FLAG_ON')  OutDataTypeStr=uint8  mask(TL_Constant){data={'output',{'variable','RTE_DEFINES/KB8_ALGO_FLAG_ON'},'date',736811.34262912034}}
      settings: DeleteFcn=if exist('delete_tlblock','file')==2,delete_tlblock(gcbh);end  NameChangeFcn=if exist('rename_tlblock','file')==2,rename_tlblock(gcbh);end  OpenFcn=if exist('tl_open_blockdlg','file')==2,tl_open_blockdlg(gcbh);else,open_system(gcbh,'parameter');end
      mask Help: eval(['if exist(''tl_online_help'',''file'') == 2, tl_online_help(''Topic'',''TL_Constant''),else, web([''jar:file:///'',matlabroot,''/help/toolbox/simulink/help.jar!/slref/' lower(get_param(gcbh,'Blocktype')) '.html''], ''-helpbrowser''),end'])
      mask Display: plot([-0.05, 1.05, NaN, -0.05, 1.05],[.01, .01, NaN, .99, .99])
  Out : Outport  PortDimensions=1  InitialOutput=[0]
  wires:
  Constant1/1 -> Out/1

== system PRO_TestHarness/PRO_AC_ProductionCycles/Subsystem/PRO_AC_ProductionCycles/PRO_AC_ProductionCycles/PRO_runProductionCycles/PRO enabled/FctTrigAbortCycle_AllPRO/For Iterator Subsystem/Algo PRO/FctTrigg_PRO/ToFormatFlag_TriggeringOrder/If Action Subsystem1 ==
  Action Port : ActionPort  ActionType=else
  Constant1 : Constant  Value=ddv('RTE_DEFINES/KB8_ALGO_FLAG_OFF')  OutDataTypeStr=uint8  mask(TL_Constant){data={'output',{'variable','RTE_DEFINES/KB8_ALGO_FLAG_OFF'},'date',736811.34272321756}}
      settings: DeleteFcn=if exist('delete_tlblock','file')==2,delete_tlblock(gcbh);end  NameChangeFcn=if exist('rename_tlblock','file')==2,rename_tlblock(gcbh);end  OpenFcn=if exist('tl_open_blockdlg','file')==2,tl_open_blockdlg(gcbh);else,open_system(gcbh,'parameter');end
      mask Help: eval(['if exist(''tl_online_help'',''file'') == 2, tl_online_help(''Topic'',''TL_Constant''),else, web([''jar:file:///'',matlabroot,''/help/toolbox/simulink/help.jar!/slref/' lower(get_param(gcbh,'Blocktype')) '.html''], ''-helpbrowser''),end'])
      mask Display: plot([-0.05, 1.05, NaN, -0.05, 1.05],[.01, .01, NaN, .99, .99])
  Out : Outport  PortDimensions=1  InitialOutput=[0]
  wires:
  Constant1/1 -> Out/1

== system PRO_TestHarness/PRO_AC_ProductionCycles/Subsystem/PRO_AC_ProductionCycles/PRO_AC_ProductionCycles/PRO_runProductionCycles/PRO enabled/FctTrigAbortCycle_AllPRO/For Iterator Subsystem/Algo PRO/FctTrigg_PRO/ToFormat_TriggeringSource/None ==
  Action Port : ActionPort  ActionType=else
  Constant6 : Constant  Value=ddv('RTE_DEFINES/KU8_TRIGGERING_SOURCE_NONE')  OutDataTypeStr=uint8  mask(TL_Constant){data={'output',{'variable','RTE_DEFINES/KU8_TRIGGERING_SOURCE_NONE'},'date',736811.34307922458}}
      settings: DeleteFcn=if exist('delete_tlblock','file')==2,delete_tlblock(gcbh);end  NameChangeFcn=if exist('rename_tlblock','file')==2,rename_tlblock(gcbh);end  OpenFcn=if exist('tl_open_blockdlg','file')==2,tl_open_blockdlg(gcbh);else,open_system(gcbh,'parameter');end
      mask Help: eval(['if exist(''tl_online_help'',''file'') == 2, tl_online_help(''Topic'',''TL_Constant''),else, web([''jar:file:///'',matlabroot,''/help/toolbox/simulink/help.jar!/slref/' lower(get_param(gcbh,'Blocktype')) '.html''], ''-helpbrowser''),end'])
      mask Display: plot([-0.05, 1.05, NaN, -0.05, 1.05],[.01, .01, NaN, .99, .99])
  u8TriggeringSource : Outport  PortDimensions=1
  wires:
  Constant6/1 -> u8TriggeringSource/1

== system PRO_TestHarness/PRO_AC_ProductionCycles/Subsystem/PRO_AC_ProductionCycles/PRO_AC_ProductionCycles/PRO_runProductionCycles/PRO enabled/FctTrigAbortCycle_AllPRO/For Iterator Subsystem/Algo PRO/FctTrigg_PRO/ToFormat_TriggeringSource/Tester ==
  Action Port : ActionPort  ActionType=then
  Constant6 : Constant  Value=ddv('RTE_DEFINES/KU8_TRIGGERING_SOURCE_TESTER')  OutDataTypeStr=uint8  mask(TL_Constant){data={'output',{'variable','RTE_DEFINES/KU8_TRIGGERING_SOURCE_TESTER'},'date',736811.34296126163}}
      settings: DeleteFcn=if exist('delete_tlblock','file')==2,delete_tlblock(gcbh);end  NameChangeFcn=if exist('rename_tlblock','file')==2,rename_tlblock(gcbh);end  OpenFcn=if exist('tl_open_blockdlg','file')==2,tl_open_blockdlg(gcbh);else,open_system(gcbh,'parameter');end
      mask Help: eval(['if exist(''tl_online_help'',''file'') == 2, tl_online_help(''Topic'',''TL_Constant''),else, web([''jar:file:///'',matlabroot,''/help/toolbox/simulink/help.jar!/slref/' lower(get_param(gcbh,'Blocktype')) '.html''], ''-helpbrowser''),end'])
      mask Display: plot([-0.05, 1.05, NaN, -0.05, 1.05],[.01, .01, NaN, .99, .99])
  u8TriggeringSource : Outport  PortDimensions=1
  wires:
  Constant6/1 -> u8TriggeringSource/1
